simulink model "AsteroidImpact"  (R2020a)
settings: Solver=ode4  StartTime=0.0  StopTime=45  FixedStep=0.1  RelTol=1e-3
values from neighbouring files (symbols this model uses):
  K = lqr(A, B, Q, R)    [rocket_dynamics.m]
settings Model: Creator=KNMALE002  LastModifiedBy=jason
settings DataIOCC: SaveOutput=off  SignalLogging=off  DSMLogging=off  ReturnWorkspaceOutputs=off  TimeSaveName=simulation_time
settings DebuggingCC: ArithmeticOperatorsInVariantConditions=warning
settings SFSimCC: CustomCodeUndefinedFunction=UseInterfaceOnly

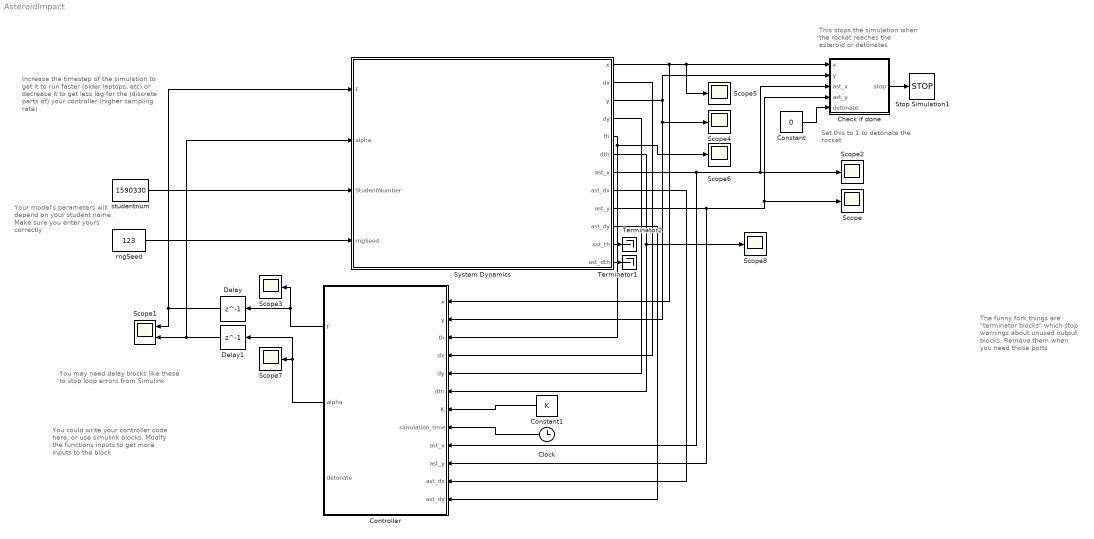
== system AsteroidImpact ==
  note: Increase the timestep of the simulation to get it to run faster (older laptops, etc) or decrease it to get less lag for the (discrete parts of) your controller (higher sampling rate)
  note: You may need delay blocks like these to stop loop errors from Simulink
  note: Your model's parameters will depend on your student name. Make sure you enter yours correctly
  note: You could write your controller code here, or use simulink blocks. Modify the functions inputs to get more inputs to the block
  note: The funny fork things are "terminator blocks" which stop warnings about unused output blocks. Remove them when you need those ports
  note: This stops the simulation when the rocket reaches the asteroid or detonates
  note: Set this to 1 to detonate the rocket
  Check if done : MATLAB Function  TreatAsAtomicUnit=on
  Clock : Clock
  Constant : Constant  Value=0
  Constant1 : Constant  Value=K
  Controller : MATLAB Function  TreatAsAtomicUnit=on
  Delay : Delay  DelayLength=1  InitialCondition=10000000
  Delay1 : Delay  DelayLength=1  InitialCondition=0.00000001
  Scope{,2..8} (8 alike) : Scope
  Scope1 : Scope  NumInputPorts=2
  Stop Simulation1 : Stop
  System Dynamics : Subsystem  TreatAsAtomicUnit=on  mask{Value=2}
      mask prompts: Value "Enter mode (1, 2 or 3)"
      mask TypeOptions Value: ScenarioVar/Value
      mask Display: image('lander.jpg');
  Terminator1 : Terminator
  Terminator2 : Terminator
  rngSeed : Constant  Value=123
  studentnum : Constant  Value=1590330
  wires:
  studentnum/1 -> System Dynamics/3(StudentNumber)
  System Dynamics/1(x) -> Scope5/1, Check if done/1(x), Controller/1(x)
  rngSeed/1 -> System Dynamics/4(rngSeed)
  System Dynamics/3(y) -> Check if done/2(y), Scope4/1, Controller/2(y)
  System Dynamics/7(ast_x) -> Controller/9(ast_x), Scope2/1, Check if done/3(ast_x)
  System Dynamics/9(ast_y) -> Controller/10(ast_y), Scope/1, Check if done/4(ast_y)
  Check if done/1(stop) -> Stop Simulation1/1
  Delay1/1 -> System Dynamics/2(alpha), Scope1/2
  Delay/1 -> System Dynamics/1(F), Scope1/1
  Controller/1(F) -> Scope3/1, Delay/1
  Controller/2(alpha) -> Delay1/1, Scope7/1
  System Dynamics/4(dy) -> Controller/5(dy)
  System Dynamics/5(th) -> Scope6/1, Controller/3(th)
  System Dynamics/2(dx) -> Controller/4(dx)
  System Dynamics/6(dth) -> Scope8/1, Controller/6(dth)
  System Dynamics/11(ast_th) -> Terminator2/1
  System Dynamics/12(ast_dth) -> Terminator1/1
  Constant1/1 -> Controller/7(K)
  Clock/1 -> Controller/8(simulation_time)
  System Dynamics/8(ast_dx) -> Controller/11(ast_dx)
  System Dynamics/10(ast_dy) -> Controller/12(ast_dy)
  Constant/1 -> Check if done/5(detonate)

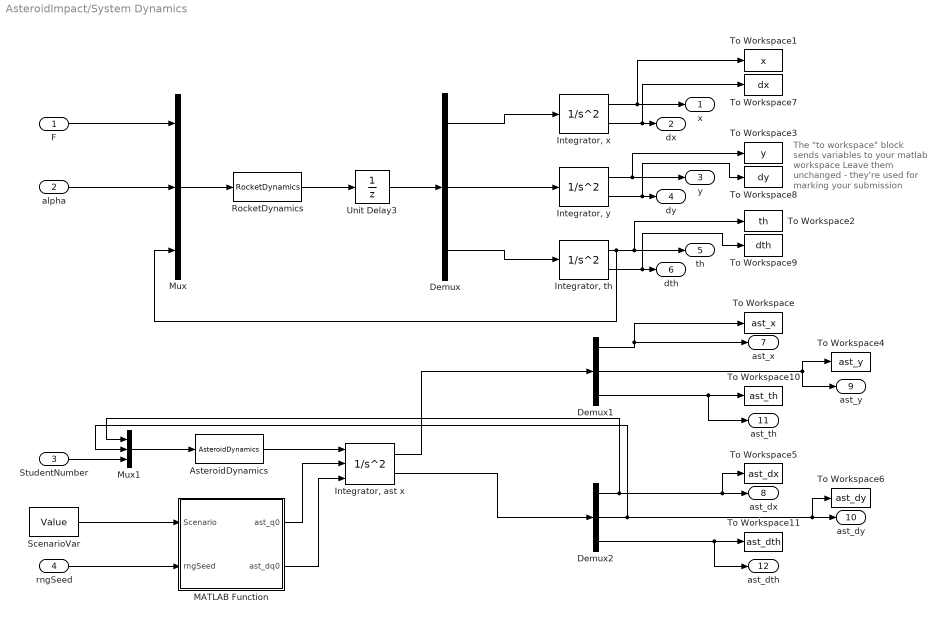
== system AsteroidImpact/System Dynamics ==
  note: The "to workspace" block sends variables to your matlab workspace
      |
      | Leave them unchanged - they're used for marking your submission
  F : Inport
  alpha : Inport  Port=2
  StudentNumber : Inport  Port=3
  rngSeed : Inport  Port=4
  AsteroidDynamics : MATLABFcn  MATLABFcn=AsteroidDynamics  OutputDimensions=3
  Demux : Demux  Outputs=3
  Demux1 : Demux  Outputs=3
  Demux2 : Demux  Outputs=3
  "Integrator, th" : SecondOrderIntegrator  ICX=0  ICDXDT=0
  "Integrator, x" : SecondOrderIntegrator  ICX=0
  "Integrator, y" : SecondOrderIntegrator  ICX=0
  "Integrator, ast x" : SecondOrderIntegrator  ICSourceX=external  ICX=x0  ICSourceDXDT=external
  MATLAB Function : MATLAB Function  TreatAsAtomicUnit=on
  Mux : Mux  Inputs=3
  Mux1 : Mux  Inputs=3
  RocketDynamics : MATLABFcn  MATLABFcn=RocketDynamics  Output1D=off
  ScenarioVar : Constant  Value=Value
  To Workspace : ToWorkspace  VariableName=ast_x  SampleTime=-1
  To Workspace1 : ToWorkspace  VariableName=x  SampleTime=-1
  To Workspace10 : ToWorkspace  VariableName=ast_th  SampleTime=-1
  To Workspace11 : ToWorkspace  VariableName=ast_dth  SampleTime=-1
  To Workspace2 : ToWorkspace  VariableName=th  SampleTime=-1
  To Workspace3 : ToWorkspace  VariableName=y  SampleTime=-1
  To Workspace4 : ToWorkspace  VariableName=ast_y  SampleTime=-1
  To Workspace5 : ToWorkspace  VariableName=ast_dx  SampleTime=-1
  To Workspace6 : ToWorkspace  VariableName=ast_dy  SampleTime=-1
  To Workspace7 : ToWorkspace  VariableName=dx  SampleTime=-1
  To Workspace8 : ToWorkspace  VariableName=dy  SampleTime=-1
  To Workspace9 : ToWorkspace  VariableName=dth  SampleTime=-1
  Unit Delay3 : UnitDelay  SampleTime=-1  HasFrameUpgradeWarning=on
  x : Outport  PortDimensions=1  VectorParamsAs1DForOutWhenUnconnected=off
  dx : Outport  Port=2  PortDimensions=1  VectorParamsAs1DForOutWhenUnconnected=off
  y : Outport  Port=3  PortDimensions=1  VectorParamsAs1DForOutWhenUnconnected=off
  dy : Outport  Port=4  PortDimensions=1  VectorParamsAs1DForOutWhenUnconnected=off
  th : Outport  Port=5  PortDimensions=1  VectorParamsAs1DForOutWhenUnconnected=off
  dth : Outport  Port=6  PortDimensions=1  VectorParamsAs1DForOutWhenUnconnected=off
  ast_x : Outport  Port=7  PortDimensions=1  VectorParamsAs1DForOutWhenUnconnected=off
  ast_dx : Outport  Port=8  PortDimensions=1  VectorParamsAs1DForOutWhenUnconnected=off
  ast_y : Outport  Port=9  PortDimensions=1  VectorParamsAs1DForOutWhenUnconnected=off
  ast_dy : Outport  Port=10  PortDimensions=1  VectorParamsAs1DForOutWhenUnconnected=off
  ast_th : Outport  Port=11  PortDimensions=1  VectorParamsAs1DForOutWhenUnconnected=off
  ast_dth : Outport  Port=12  PortDimensions=1  VectorParamsAs1DForOutWhenUnconnected=off
  wires:
  "Integrator, th"/1 -> th/1, To Workspace2/1, Mux/3
  Demux/1 -> "Integrator, x"/1
  Demux/2 -> "Integrator, y"/1
  Demux/3 -> "Integrator, th"/1
  "Integrator, x"/1 -> x/1, To Workspace1/1
  "Integrator, x"/2 -> To Workspace7/1, dx/1
  "Integrator, y"/2 -> To Workspace8/1, dy/1
  "Integrator, th"/2 -> To Workspace9/1, dth/1
  Mux/1 -> RocketDynamics/1
  RocketDynamics/1 -> Unit Delay3/1
  rngSeed/1 -> MATLAB Function/2(rngSeed)
  ScenarioVar/1 -> MATLAB Function/1(Scenario)
  F/1 -> Mux/1
  alpha/1 -> Mux/2
  Demux1/2 -> To Workspace4/1, ast_y/1
  Demux1/3 -> To Workspace10/1, ast_th/1
  Demux2/3 -> ast_dth/1, To Workspace11/1
  Mux1/1 -> AsteroidDynamics/1
  AsteroidDynamics/1 -> "Integrator, ast x"/1
  "Integrator, ast x"/1 -> Demux1/1
  "Integrator, ast x"/2 -> Demux2/1
  Demux1/1 -> To Workspace/1, ast_x/1
  Demux2/1 -> Mux1/1, To Workspace5/1, ast_dx/1
  Demux2/2 -> Mux1/2, To Workspace6/1, ast_dy/1
  MATLAB Function/1(ast_q0) -> "Integrator, ast x"/2
  MATLAB Function/2(ast_dq0) -> "Integrator, ast x"/3
  StudentNumber/1 -> Mux1/3
  Unit Delay3/1 -> Demux/1
  "Integrator, y"/1 -> y/1, To Workspace3/1

== matlab function AsteroidImpact/System Dynamics/MATLAB Function ==
  data: ast_q0 output; ast_dq0 output; Scenario input; rngSeed input
function [ast_q0, ast_dq0] = fcn(Scenario, rngSeed)
rng(rngSeed);

if (Scenario == 1)
    x0 = -3000;
    y0 =  5000;
    th0 =   0;
    dx0 = 182;
    dy0 = 0;
    dth0 = 0;

elseif (Scenario == 2)
    x0 = -2000 + rand_within_plus_minus(100);
    y0 = 4000 + rand_within_plus_minus(100); 
    th0 = 0;
    dx0 = 170;
    dy0 = 0;
    dth0 = 0.1;

elseif (Scenario == 3)
    x0 = -2500;
    y0 = 3000;
    th0 = 0;
    dx0 = 160;
    dy0 = 100;
    dth0 = deg2rad(rand_within_plus_minus(20)); % rad/sec

else
    error('You entered an invalid mode -- make sure Scenario = 1, 2 or 3')
end

ast_q0  = [ x0;  y0;  th0];
ast_dq0 = [dx0; dy0; dth0];

end

% calling rand_within_plus_minus(100) returns a number between -100 and 100
function n = rand_within_plus_minus(interval)
    n = (rand - 0.5) * 2 * interval;
end

== matlab function AsteroidImpact/Controller ==
  data: x input; F output; alpha output; y input; th input; dx input; dy input; dth input; K input; simulation_time input; ast_x input; ast_y input; detonate output; ast_dx input; ast_dy input
function [F, alpha, detonate] = fcn(x, y, th, dx, dy, dth, K, simulation_time, ast_x, ast_y, ast_dx, ast_dy)

if (abs(ast_x - x) < 80 && abs(ast_y - y) < 80)
    detonate = 1;
else
    detonate = 0;
end

% x_target = x - 1000;
% y_target = y - 2500;
% 
% linpoint = [dx; dy; dth*30; x_target; y_target; th*10];
% 
% linpoint = K*linpoint;
% 
% ctrlInput = [1000*9.81; 0] - linpoint;
% Fout = ctrlInput(1);
% alphaout = ctrlInput(2);
% 
% if Fout > 36000 
%    Fout = 36000;
% elseif Fout < 0
%     Fout = 1000*9.81/2;
% end
% 
% F = Fout;
% alpha = 0.001*alphaout; %alphaout;

% Direct Rocket
% if x < 1500
%     x_target = x - 1500;
%     y_target = y - 1500;
% else
%     x_target = x - ast_x;
%     y_target = y - ast_y;
% end

% Prevent over-dominance of x weighting at the beginning
% if abs(x_target) > 500
%     K(2,4) = 0.5*K(2,4);
% end

% if simulation_time < 3
%     if alphaout > 0.1 
%        alphaout = 0.1;
%     elseif alphaout < -0.1
%        alphaout = -0.1;
%     end
% else
%     if alphaout > 1.5 
%        alphaout = 1.5;
%     elseif alphaout < -1.5
%        alphaout = -1.5;
%     end
% end

% Over Turn recovery
% if th > pi/4
%     Fout = 1000*9.81;
%     alphaout = pi/2;
% elseif th < -pi/4
%     Fout = 1000*9.81;
%     alphaout = -pi/2;
% end

% INERTIAL INTERCEPT LQR

R = [ast_x; ast_y] - [x; y];
Rtemp = [R; 0];
Vr = [ast_dx; ast_dy] - [dx; dy];
Vtemp = [Vr; 0];
omega = cross(Rtemp, Vtemp) / dot(Rtemp, Rtemp);
temp = cross(Vtemp, omega);
aN = 20*temp(1:2);

vN = aN.*simulation_time;
vN(1,1) = vN(1,1);
vN(2,1) = vN(2,1);
vN = vN - [dx; dy];

inp = K(:,3:4)*vN + [1000*9.81; 0] - (K(:,1:2)*[th - 0; dth - 0]);
Fout = inp(1);
alphaout = inp(2);

if Fout > 36000 
   Fout = 36000;
elseif Fout < 0
    Fout = 0;
end

if alphaout > 1.5 
   alphaout = 1.5;
elseif alphaout < -1.5
    alphaout = -1.5;
end

F = Fout;
alpha = alphaout;

== matlab function AsteroidImpact/Check if done ==
  data: x input; stop output; y input; ast_x input; ast_y input; detonate input
function stop = fcn(x, y, ast_x, ast_y, detonate)
    % given the signal to detonate
    if detonate == 1
        stop = 1;

    % rocket has hit the asteroid
    elseif norm([x; y] - [ast_x; ast_y]) < 100
        stop = 1;
    
    % rocket has hit the ground OR asteroid is close to they city
    elseif y < 0 || ast_y < 200
        stop = 1;
    
    else
        stop = 0;
    end
end
